simulink model "simulator_Force_Model"  (R2025b)
settings: Solver=FixedStepAuto  StartTime=0.0  StopTime=80  FixedStep=0.01  RelTol=1e-3
values from neighbouring files (symbols this model uses):
  dt = system_params.dt    [discretize_system.m]    (also in model_init.m)
  q0 = [0; 0; 0]    [model_init.m]    (also in test_model.m = x_test(1:3))
  qdot0 = [0;0;0]    [model_init.m]
undefined symbols (not defined in the file or in its folder): Cd, Dd, EKF_settings, P0, system_params, x0_EKF
libraries: slpidlib x5, mpclib x2
settings Model: Creator=Sigbjørn  LastModifiedBy=sig

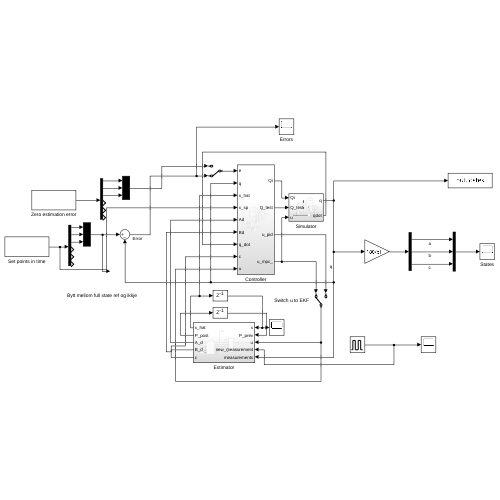
[thumbnail: Simulink's stored preview of the top-level diagram]
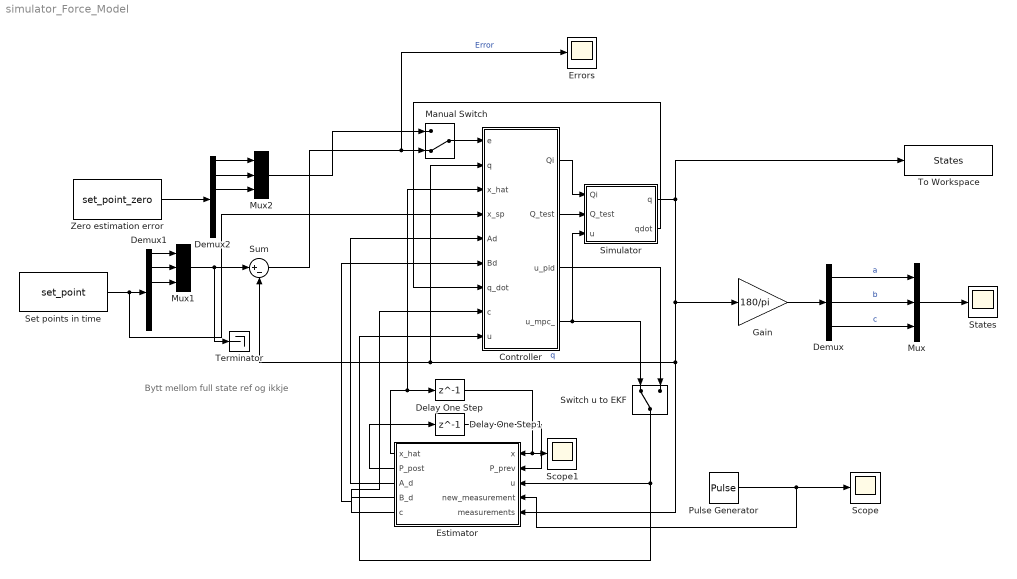
== system simulator_Force_Model ==
  note: Bytt mellom full state ref og ikkje
  Controller : Subsystem
  Delay One Step : Delay  DelayLength=1  InitialCondition=x0_EKF
  Delay One Step1 : Delay  DelayLength=1  InitialCondition=P0
  Demux : Demux  Outputs=3
  Demux1 : Demux  Outputs=6
  Demux2 : Demux  Outputs=6
  Errors : Scope
      settings: ActiveDisplayYMinimum=-1.818734816898053E+64  ActiveDisplayYMaximum=2.7677532819561327E+63
  Estimator : Subsystem
      settings: PortSchema="{\"entries\":[{\"content\":{\"sides\":[{\"content\":{\"connectorIds\":[\"Out1\",\"Out2\",\"Out3\",\"Out4\",\"Out5\"]},\"type\":\"ConnectorPlacement.EquallySpacedRectSide\",\"uuid\":\"f477ef40-4352-4d84-a45f-d7b8149414e1\"},{\"content\":{\"connectorIds\":[\"In1\",\"In2\",\"In3\",\"In4\",\"In5\"],\"side\":\"RIGHT\"},\"type\":\"ConnectorPlacement.EquallySpacedRectSide\",\"uuid\":\"8f29c47b-7819-47b7-a7db-3d460012710f\"},{\"content\":{\"side\":\"TOP\"},\"type\":\"ConnectorPlacement.EquallySpacedRectSide\",\"uuid\":\"6fcef62b-5cfa-49ba-93f4-5d540223ca0d\"}]},\"type\":\"ConnectorPlacement.EquallySpacedConnector\",\"uuid\":\"aa31ebfc-db05-4e23-be25-e9e271d34221\"}],\"packageUris\":[\"http://schema.mathworks.com/mf0/Connector/R2020b\"],\"version\":\"1.0\"}"
  Gain : Gain  Gain=180/pi
  Manual Switch : ManualSwitch  CurrentSetting=0
  Mux : Mux  Inputs=3
  Mux1 : Mux  Inputs=3
  Mux2 : Mux  Inputs=3
  Pulse Generator : DiscretePulseGenerator  PulseType=Time based  Period=0.02  PulseWidth=50
  Scope : Scope
      settings: ActiveDisplayYMinimum=-0.12120060790273554  ActiveDisplayYMaximum=1.1287993920972645  DataLoggingVariableName=ScopeData11
  Scope1 : Scope
      settings: ActiveDisplayYMinimum=-0.06497104688761951  ActiveDisplayYMaximum=0.02165522822111654  DataLoggingVariableName=ScopeData13
  Set points in time : FromWorkspace  VariableName=set_point
  Simulator : Subsystem
  States : Scope
      settings: ActiveDisplayYMinimum=-31.388895783470453  ActiveDisplayYMaximum=57.369364436172283
  Sum : Sum  Inputs=|+-
  Switch u to EKF : ManualSwitch
  Terminator : Terminator
  To Workspace : ToWorkspace  VariableName=States  SaveFormat=Timeseries  SampleTime=-1
  Zero estimation error : FromWorkspace  VariableName=set_point_zero
  wires:
  Controller/1(Qi) -> Simulator/1(Qi)
  Sum/1 -> Errors/1, Manual Switch/2  "Error"
  Simulator/1(q) -> To Workspace/1, Estimator/5(measurements), Sum/2, Controller/2(q), Gain/1  "q"
  Demux/1 -> Mux/1  "a"
  Demux/2 -> Mux/2  "b"
  Demux/3 -> Mux/3  "c"
  Manual Switch/1 -> Controller/1(e)
  Gain/1 -> Demux/1
  Mux/1 -> States/1
  Controller/2(Q_test) -> Simulator/2(Q_test)
  Pulse Generator/1 -> Estimator/4(new_measurement), Scope/1
  Estimator/2(P_post) -> Delay One Step1/1
  Delay One Step/1 -> Scope1/1, Estimator/1(x)
  Delay One Step1/1 -> Estimator/2(P_prev)
  Estimator/3(A_d) -> Controller/5(Ad)
  Estimator/4(B_d) -> Controller/6(Bd)
  Demux1/2 -> Mux1/2
  Demux1/1 -> Mux1/1
  Demux1/3 -> Mux1/3
  Mux1/1 -> Terminator/1, Sum/1
  Estimator/1(x_hat) -> Controller/3(x_hat), Delay One Step/1
  Demux2/3 -> Mux2/3
  Demux2/2 -> Mux2/2
  Zero estimation error/1 -> Demux2/1
  Demux2/1 -> Mux2/1
  Mux2/1 -> Manual Switch/1
  Simulator/2(qdot) -> Controller/7(q_dot)
  Estimator/5(c) -> Controller/8(c)
  Switch u to EKF/1 -> Estimator/3(u), Controller/9(u)
  Controller/4(u_mpc_) -> Switch u to EKF/1, Simulator/3(u)
  Controller/3(u_pid) -> Switch u to EKF/2
  Set points in time/1 -> Controller/4(x_sp), Demux1/1

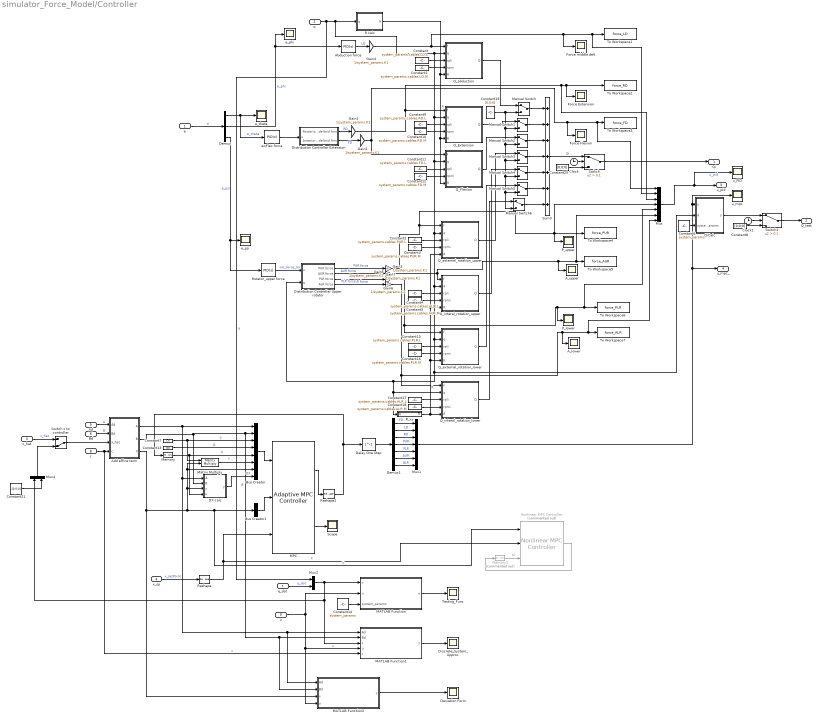
== system simulator_Force_Model/Controller ==
  e : Inport
  q : Inport  Port=2
  x_hat : Inport  Port=3
  x_sp : Inport  Port=4
  Ad : Inport  Port=5
  Bd : Inport  Port=6
  q_dot : Inport  Port=7
  c : Inport  Port=8
  u : Inport  Port=9
  A_lower : Scope
      settings: ActiveDisplayYMinimum=-66.70773  ActiveDisplayYMaximum=600.36959  DataLoggingVariableName=ScopeData3
  A_upper : Scope
      settings: ActiveDisplayYMinimum=-10.373094653487385  ActiveDisplayYMaximum=93.35785188138648  DataLoggingVariableName=ScopeData4
  Abduction force : slpidlib/PID Controller  Controller=PID  Form=Parallel  TimeDomain=Continuous-time  UseExternalTs=off  SampleTime=-1  IntegratorMethod=Forward Euler  FilterMethod=Forward Euler  ControllerParametersSource=internal  P=1  I=25  UseKiTs=off  D=5  UseExternalDerivativeSource=off  N=100  UseFilter=on  TunerSelectOption=Transfer Function Based (PID Tuner App)  InitialConditionSource=internal  InitialConditionForIntegrator=0  InitialConditionForFilter=0  DifferentiatorICPrevScaledInput=0  ExternalReset=none  TrackingMode=off  Kt=1  LimitOutput=on  SatLimitsSource=internal  UpperSaturationLimit=inf  LowerSaturationLimit=0  LinearizeAsGain=on  AntiWindupMode=none  Kb=1  LimitIntegrator=on  UpperIntegratorSaturationLimit=10000  LowerIntegratorSaturationLimit=0  POutMin=[]  POutMax=[]  IOutMin=[]  IOutMax=[]  DOutMin=[]  DOutMax=[]  NOutMin=[]  NOutMax=[]  SumOutMin=[]  SumOutMax=[]  SaturationOutMin=[]  SaturationOutMax=[]  PParamMin=[]  PParamMax=[]  IParamMin=[]  IParamMax=[]  DParamMin=[]  DParamMax=[]  NParamMin=[]  NParamMax=[]  KbParamMin=[]  KbParamMax=[]  KtParamMin=[]  KtParamMax=[]  KbOutMin=[]  KbOutMax=[]  KtOutMin=[]  KtOutMax=[]  IntegratorOutMin=[]  IntegratorOutMax=[]  FilterOutMin=[]  FilterOutMax=[]  SumI1OutMin=[]  SumI1OutMax=[]  SumI2OutMin=[]  SumI2OutMax=[]  SumI3OutMin=[]  SumI3OutMax=[]  SumI4OutMin=[]  SumI4OutMax=[]  SumDOutMin=[]  SumDOutMax=[]  DifferentiatorOutMin=[]  DifferentiatorOutMax=[]  FilterDiffOutCoefMin=[]  FilterDiffOutCoefMax=[]  ReciprocalOutMin=[]  ReciprocalOutMax=[]  SumDenOutMin=[]  SumDenOutMax=[]  SumNumOutMin=[]  SumNumOutMax=[]  DivideOutMin=[]  DivideOutMax=[]  UdiffTsProdOutMin=[]  UdiffTsProdOutMax=[]  NTsProdOutMin=[]  NTsProdOutMax=[]  UintegralTsProdOutMin=[]  UintegralTsProdOutMax=[]  UngainTsProdOutMin=[]  UngainTsProdOutMax=[]  ClampingZeroOutDataTypeStr=Inherit: Inherit via back propagation  ClampingZeroOutMin=[]  ClampingZeroOutMax=[]  FilterDenConstantOutDataTypeStr=Inherit: Inherit via back propagation  FilterDenConstantOutMin=[]  FilterDenConstantOutMax=[]  PCopyOutDataTypeStr=Inherit: Inherit via back propagation  PCopyOutMin=[]  PCopyOutMax=[]  NCopyOutDataTypeStr=Inherit: Inherit via back propagation  NCopyOutMin=[]  NCopyOutMax=[]  IntegratorContinuousStateAttributes=''  IntegratorStateMustResolveToSignalObject=off  IntegratorRTWStateStorageClass=Auto  FilterContinuousStateAttributes=''  FilterStateMustResolveToSignalObject=off  FilterRTWStateStorageClass=Auto  ParallelPVariant=InternalParameters  IdealPVariant=Disabled  IVariant=InternalParameters  DVariant=InternalParameters  IntegratorVariant=Continuous  SatVariant=Enabled  AWVariant=Passthrough  PCopyVariant=Disabled  TRVariant=Disabled  FdbkBlocksVariant=Forward  IdealPFdbkVariant=Disabled  SatFdbkVariant=Disabled  DerivativeFilterVariant=ContFilter  NVariant=InternalParameters  NCopyVariant=Disabled  FilterICVariant=InternalICsFilter  IntegratorICVariant=InternalICs  ExternalResetVariant=Disabled  TRSumVariant=Passthrough  SumFdbkVariant=Disabled  SumVariant=Sum_PID  TsampFilterVariant=InternalTs  TsampNgainVariant=Passthrough  TsampIntegralVariant=Disabled_SignalSpec  ExternalSaturationOutDataTypeStr=Inherit: Same as second input  DerivativeSourceVariant=ErrorSignal  PreIntVariant=InternalPreInt
  Add affine term : MATLAB Function  TreatAsAtomicUnit=on
  Bus Creator : BusCreator  Inputs=8
  Bus Creator1 : BusCreator  Inputs=1
  Clock : Clock
  Clock1 : Clock
  Constant : Constant  Value=system_params.cables.LD.L
  Constant1 : Constant  Value=system_params.cables.LD.M
  Constant10 : Constant  Value=system_params.cables.RD.M
  Constant11 : Constant  Value=system_params.cables.FD.L
  Constant12 : Constant  Value=system_params.cables.FD.M
  Constant13 : Constant  Value=Dd
  Constant14 : Constant  Value=system_params  OutDataTypeStr=Bus: System_params_bus
  Constant15 : Constant  Value=system_params.cables.PLR.L
  Constant16 : Constant  Value=system_params.cables.PLR.M
  Constant17 : Constant  Value=system_params.cables.ALR.L
  Constant18 : Constant  Value=system_params.cables.ALR.M
  Constant{8,19,21,25} (4 alike) : Constant  Value=[0;0;0]
  Constant2 : Constant  Value=system_params.cables.PUR.L
  Constant3 : Constant  Value=system_params.cables.PUR.M
  Constant4 : Constant  Value=system_params.cables.AUR.L
  Constant5 : Constant  Value=system_params.cables.AUR.M
  Constant6 : Constant  Value=system_params  OutDataTypeStr=Bus: System_params_bus
  Constant7 : Constant  Value=Cd
  Constant9 : Constant  Value=system_params.cables.RD.L
  DX calc : MATLAB Function  TreatAsAtomicUnit=on
  Delay One Step : Delay  DelayLength=1
  Demux : Demux  Outputs=3
  Demux1 : Demux  Outputs=7
  Deviation Form : Scope
      settings: ActiveDisplayYMinimum=-1  ActiveDisplayYMaximum=1  DataLoggingVariableName=ScopeData20
  Discrete_System_Approx : Scope
      settings: ActiveDisplayYMinimum=-0.51528443829155268  ActiveDisplayYMaximum=1.8768209864297223  DataLoggingVariableName=ScopeData18
  Distribution Controller Extension : Subsystem
  Distribution Controller Upper rotator : Subsystem
  Force Extension : Scope
      settings: ActiveDisplayYMinimum=-1.1404457548759319E-5  ActiveDisplayYMaximum=0.0001033020677424701
  Force Flexion : Scope
      settings: ActiveDisplayYMinimum=-0.00021802888941381923  ActiveDisplayYMaximum=0.0019628886422166426  DataLoggingVariableName=ScopeData2
  Force middle delt : Scope
      settings: ActiveDisplayYMinimum=-0.45342522545906838  ActiveDisplayYMaximum=4.0808270291316164  DataLoggingVariableName=ScopeData3
  Gain{1..7} (7 alike) : Gain  Gain=1/system_params.K1
  MATLAB Function : MATLAB Function  TreatAsAtomicUnit=on
  MATLAB Function1 : MATLAB Function  TreatAsAtomicUnit=on
  MATLAB Function2 : MATLAB Function  TreatAsAtomicUnit=on
  MPC : mpclib/Adaptive MPC Controller  SCDEnableBlockLinearizationSpecification=on  mpcobj=MPC_controller  enable_value=0  updateMPCinCallerWorkspace=on  md_inport=off  mv_inport=off  uref_inport=off  return_cost=on  return_mvseq=off  return_qpstatus=off  return_xseq=off  return_state=off  return_ovseq=off  state_inport=on  isltv_plant=off  umin_inport=off  umax_inport=off  ymin_inport=off  ymax_inport=off  cc_inport=off  ywt_inport=off  uwt_inport=off  duwt_inport=off  rhoeps_inport=off  pm_inport=off  MaximumP=10  HorizonChoice=FixedHorizon  BlockDataType=double  SampleTimeInherited=off  switch_inport=off
  Manual Switch{,1..6} (7 alike) : ManualSwitch
  Matrix Multiply : Product  Multiplication=Matrix(*)
  Memory : Memory  InitialCondition=[0;0;0;0;0;0;0]
  Memory1 : Memory  Commented=on  InitialCondition=[0;0;0;0;0;0;0]
  Mux : Mux  Inputs=7
  Mux1 : Mux  Inputs=7
  Mux2 : Mux  Inputs=2
  Mux4 : Mux  Inputs=2
  Nonlinear MPC Controller : mpclib/Nonlinear MPC Controller  Commented=on  nlmpcobj=NL_mpc  UseObjectTs=on  UseMEX=off  md_enabled=off  mvtarget_enabled=off  param_enabled=off  cost_enabled=off  mvseq_enabled=off  stateseq_enabled=off  ovseq_enabled=off  slack_enabled=off  status_enabled=off  ov_min=off  ov_max=off  mv_min=off  mv_max=off  mvrate_min=off  mvrate_max=off  state_min=off  state_max=off  ov_weight=off  mv_weight=off  mvrate_weight=off  ecr_weight=off  nlp_initialize=off
  P_lower : Scope
      settings: ActiveDisplayYMinimum=-3.51093  ActiveDisplayYMaximum=31.5984  DataLoggingVariableName=ScopeData2
  P_upper : Scope
      settings: ActiveDisplayYMinimum=-0.42649  ActiveDisplayYMaximum=3.83839
  Q_Extension : MATLAB Function  TreatAsAtomicUnit=on
  Q_Flexion : MATLAB Function  TreatAsAtomicUnit=on
  Q_abduction : MATLAB Function  TreatAsAtomicUnit=on
  Q_external_rotation_lower : MATLAB Function  TreatAsAtomicUnit=on
  Q_external_rotation_upper : MATLAB Function  TreatAsAtomicUnit=on
  Q_interal_rotation_lower : MATLAB Function  TreatAsAtomicUnit=on
  Q_interal_rotation_upper : MATLAB Function  TreatAsAtomicUnit=on
  QiCalc : MATLAB Function  TreatAsAtomicUnit=on
  R calc : MATLAB Function  TreatAsAtomicUnit=on
  R_xy : MATLAB Function  TreatAsAtomicUnit=on
  Reshape : Reshape  OutputDimensionality=Column vector (2-D)
  Reshape1 : Reshape  OutputDimensionality=Column vector (2-D)
  Rotator_upper force : slpidlib/PID Controller  Controller=PID  Form=Parallel  TimeDomain=Continuous-time  UseExternalTs=off  SampleTime=-1  IntegratorMethod=Forward Euler  FilterMethod=Forward Euler  ControllerParametersSource=internal  P=100  I=200  UseKiTs=off  D=500  UseExternalDerivativeSource=off  N=100  UseFilter=on  TunerSelectOption=Transfer Function Based (PID Tuner App)  InitialConditionSource=internal  InitialConditionForIntegrator=0  InitialConditionForFilter=0  DifferentiatorICPrevScaledInput=0  ExternalReset=none  TrackingMode=off  Kt=1  LimitOutput=on  SatLimitsSource=internal  UpperSaturationLimit=inf  LowerSaturationLimit=-inf  LinearizeAsGain=on  AntiWindupMode=none  Kb=1  LimitIntegrator=on  UpperIntegratorSaturationLimit=inf  LowerIntegratorSaturationLimit=-inf  POutMin=[]  POutMax=[]  IOutMin=[]  IOutMax=[]  DOutMin=[]  DOutMax=[]  NOutMin=[]  NOutMax=[]  SumOutMin=[]  SumOutMax=[]  SaturationOutMin=[]  SaturationOutMax=[]  PParamMin=[]  PParamMax=[]  IParamMin=[]  IParamMax=[]  DParamMin=[]  DParamMax=[]  NParamMin=[]  NParamMax=[]  KbParamMin=[]  KbParamMax=[]  KtParamMin=[]  KtParamMax=[]  KbOutMin=[]  KbOutMax=[]  KtOutMin=[]  KtOutMax=[]  IntegratorOutMin=[]  IntegratorOutMax=[]  FilterOutMin=[]  FilterOutMax=[]  SumI1OutMin=[]  SumI1OutMax=[]  SumI2OutMin=[]  SumI2OutMax=[]  SumI3OutMin=[]  SumI3OutMax=[]  SumI4OutMin=[]  SumI4OutMax=[]  SumDOutMin=[]  SumDOutMax=[]  DifferentiatorOutMin=[]  DifferentiatorOutMax=[]  FilterDiffOutCoefMin=[]  FilterDiffOutCoefMax=[]  ReciprocalOutMin=[]  ReciprocalOutMax=[]  SumDenOutMin=[]  SumDenOutMax=[]  SumNumOutMin=[]  SumNumOutMax=[]  DivideOutMin=[]  DivideOutMax=[]  UdiffTsProdOutMin=[]  UdiffTsProdOutMax=[]  NTsProdOutMin=[]  NTsProdOutMax=[]  UintegralTsProdOutMin=[]  UintegralTsProdOutMax=[]  UngainTsProdOutMin=[]  UngainTsProdOutMax=[]  ClampingZeroOutDataTypeStr=Inherit: Inherit via back propagation  ClampingZeroOutMin=[]  ClampingZeroOutMax=[]  FilterDenConstantOutDataTypeStr=Inherit: Inherit via back propagation  FilterDenConstantOutMin=[]  FilterDenConstantOutMax=[]  PCopyOutDataTypeStr=Inherit: Inherit via back propagation  PCopyOutMin=[]  PCopyOutMax=[]  NCopyOutDataTypeStr=Inherit: Inherit via back propagation  NCopyOutMin=[]  NCopyOutMax=[]  IntegratorContinuousStateAttributes=''  IntegratorStateMustResolveToSignalObject=off  IntegratorRTWStateStorageClass=Auto  FilterContinuousStateAttributes=''  FilterStateMustResolveToSignalObject=off  FilterRTWStateStorageClass=Auto  ParallelPVariant=InternalParameters  IdealPVariant=Disabled  IVariant=InternalParameters  DVariant=InternalParameters  IntegratorVariant=Continuous  SatVariant=Enabled  AWVariant=Passthrough  PCopyVariant=Disabled  TRVariant=Disabled  FdbkBlocksVariant=Forward  IdealPFdbkVariant=Disabled  SatFdbkVariant=Disabled  DerivativeFilterVariant=ContFilter  NVariant=InternalParameters  NCopyVariant=Disabled  FilterICVariant=InternalICsFilter  IntegratorICVariant=InternalICs  ExternalResetVariant=Disabled  TRSumVariant=Passthrough  SumFdbkVariant=Disabled  SumVariant=Sum_PID  TsampFilterVariant=InternalTs  TsampNgainVariant=Passthrough  TsampIntegralVariant=Disabled_SignalSpec  ExternalSaturationOutDataTypeStr=Inherit: Same as second input  DerivativeSourceVariant=ErrorSignal  PreIntVariant=InternalPreInt
  Scope : Scope
      settings: ActiveDisplayYMinimum=-740.0274786197964  ActiveDisplayYMaximum=6731.9872770462225  DataLoggingVariableName=ScopeData19
  Sum3 : Sum  Inputs=+++++++  InputSameDT=on  SaturateOnIntegerOverflow=on  OutDataTypeStr=Inherit: Same as first input
  Switch : Switch  Criteria=u2 > Threshold  Threshold=0.1  SaturateOnIntegerOverflow=off  InputSameDT=off
  Switch x to controller : ManualSwitch  CurrentSetting=0
  Switch1 : Switch  Criteria=u2 > Threshold  Threshold=0.1  SaturateOnIntegerOverflow=off  InputSameDT=off
  Testing_Func : Scope
      settings: ActiveDisplayYMinimum=-0.87802224801470286  ActiveDisplayYMaximum=2.0566387555111536  DataLoggingVariableName=ScopeData16
  To Workspace1 : ToWorkspace  VariableName=force_LD  SaveFormat=Timeseries  SampleTime=-1
  To Workspace2 : ToWorkspace  VariableName=force_RD  SaveFormat=Timeseries  SampleTime=-1
  To Workspace3 : ToWorkspace  VariableName=force_FD  SaveFormat=Timeseries  SampleTime=-1
  To Workspace4 : ToWorkspace  VariableName=force_PUR  SaveFormat=Timeseries  SampleTime=-1
  To Workspace5 : ToWorkspace  VariableName=force_AUR  SaveFormat=Timeseries  SampleTime=-1
  To Workspace6 : ToWorkspace  VariableName=force_PLR  SaveFormat=Timeseries  SampleTime=-1
  To Workspace7 : ToWorkspace  VariableName=force_ALR  SaveFormat=Timeseries  SampleTime=-1
  e_phi : Scope
      settings: ActiveDisplayYMinimum=-1  ActiveDisplayYMaximum=1  DataLoggingVariableName=ScopeData5
  e_psi : Scope
      settings: ActiveDisplayYMinimum=-0.000531028678053236  ActiveDisplayYMaximum=0.0043911774565179515  DataLoggingVariableName=ScopeData3
  e_theta : Scope
      settings: ActiveDisplayYMinimum=-0.0081249223165325481  ActiveDisplayYMaximum=0.0015822660919378819  DataLoggingVariableName=ScopeData6
  ex/flex force : slpidlib/PID Controller  Controller=PID  Form=Parallel  TimeDomain=Discrete-time  UseExternalTs=off  SampleTime=-1  IntegratorMethod=Forward Euler  FilterMethod=Forward Euler  ControllerParametersSource=internal  P=1  I=25  UseKiTs=off  D=5  UseExternalDerivativeSource=off  N=100  UseFilter=on  TunerSelectOption=Transfer Function Based (PID Tuner App)  InitialConditionSource=internal  InitialConditionForIntegrator=0  InitialConditionForFilter=0  DifferentiatorICPrevScaledInput=0  ExternalReset=none  TrackingMode=off  Kt=1  LimitOutput=on  SatLimitsSource=internal  UpperSaturationLimit=inf  LowerSaturationLimit=-inf  LinearizeAsGain=on  AntiWindupMode=none  Kb=1  LimitIntegrator=on  UpperIntegratorSaturationLimit=inf  LowerIntegratorSaturationLimit=-inf  POutMin=[]  POutMax=[]  IOutMin=[]  IOutMax=[]  DOutMin=[]  DOutMax=[]  NOutMin=[]  NOutMax=[]  SumOutMin=[]  SumOutMax=[]  SaturationOutMin=[]  SaturationOutMax=[]  PParamMin=[]  PParamMax=[]  IParamMin=[]  IParamMax=[]  DParamMin=[]  DParamMax=[]  NParamMin=[]  NParamMax=[]  KbParamMin=[]  KbParamMax=[]  KtParamMin=[]  KtParamMax=[]  KbOutMin=[]  KbOutMax=[]  KtOutMin=[]  KtOutMax=[]  IntegratorOutMin=[]  IntegratorOutMax=[]  FilterOutMin=[]  FilterOutMax=[]  SumI1OutMin=[]  SumI1OutMax=[]  SumI2OutMin=[]  SumI2OutMax=[]  SumI3OutMin=[]  SumI3OutMax=[]  SumI4OutMin=[]  SumI4OutMax=[]  SumDOutMin=[]  SumDOutMax=[]  DifferentiatorOutMin=[]  DifferentiatorOutMax=[]  FilterDiffOutCoefMin=[]  FilterDiffOutCoefMax=[]  ReciprocalOutMin=[]  ReciprocalOutMax=[]  SumDenOutMin=[]  SumDenOutMax=[]  SumNumOutMin=[]  SumNumOutMax=[]  DivideOutMin=[]  DivideOutMax=[]  UdiffTsProdOutMin=[]  UdiffTsProdOutMax=[]  NTsProdOutMin=[]  NTsProdOutMax=[]  UintegralTsProdOutMin=[]  UintegralTsProdOutMax=[]  UngainTsProdOutMin=[]  UngainTsProdOutMax=[]  ClampingZeroOutDataTypeStr=Inherit: Inherit via back propagation  ClampingZeroOutMin=[]  ClampingZeroOutMax=[]  FilterDenConstantOutDataTypeStr=Inherit: Inherit via back propagation  FilterDenConstantOutMin=[]  FilterDenConstantOutMax=[]  PCopyOutDataTypeStr=Inherit: Inherit via back propagation  PCopyOutMin=[]  PCopyOutMax=[]  NCopyOutDataTypeStr=Inherit: Inherit via back propagation  NCopyOutMin=[]  NCopyOutMax=[]  IntegratorContinuousStateAttributes=''  IntegratorStateMustResolveToSignalObject=off  IntegratorRTWStateStorageClass=Auto  FilterContinuousStateAttributes=''  FilterStateMustResolveToSignalObject=off  FilterRTWStateStorageClass=Auto  ParallelPVariant=InternalParameters  IdealPVariant=Disabled  IVariant=InternalParameters  DVariant=InternalParameters  IntegratorVariant=Discrete  SatVariant=Enabled  AWVariant=Passthrough  PCopyVariant=Disabled  TRVariant=Disabled  FdbkBlocksVariant=Forward  IdealPFdbkVariant=Disabled  SatFdbkVariant=Disabled  DerivativeFilterVariant=ForwardEulerFilter  NVariant=InternalParameters  NCopyVariant=Disabled  FilterICVariant=InternalICsFilter  IntegratorICVariant=InternalICs  ExternalResetVariant=Disabled  TRSumVariant=Passthrough  SumFdbkVariant=Disabled  SumVariant=Sum_PID  TsampFilterVariant=InternalTs  TsampNgainVariant=Passthrough  TsampIntegralVariant=Disabled_SignalSpec  ExternalSaturationOutDataTypeStr=Inherit: Same as second input  DerivativeSourceVariant=ErrorSignal  PreIntVariant=InternalPreInt
  u_PID : Scope
      settings: ActiveDisplayYMinimum=-0.0655807466436869  ActiveDisplayYMaximum=0.59022671979318231  DataLoggingVariableName=ScopeData15
  u_mpc : Scope
      settings: ActiveDisplayYMinimum=-0.10232300884956036  ActiveDisplayYMaximum=0.21294247787611242  DataLoggingVariableName=ScopeData14
  Qi : Outport
  Q_test : Outport  Port=2
  u_pid : Outport  Port=3
  u_mpc_ : Outport  Port=4
  wires:
  q/1 -> Mux2/1, Q_abduction/2(q), Q_Extension/2(q), Q_Flexion/2(q), QiCalc/2(q), Q_interal_rotation_lower/2(q), R_xy/1(q), Distribution Controller Upper rotator/2(q), Q_external_rotation_lower/2(q), Q_interal_rotation_upper/2(q), Q_external_rotation_upper/2(q), R calc/1(q)  "q"
  R calc/1(R) -> Q_Extension/5(R), Q_Flexion/5(R), Q_abduction/5(R)  "R"
  Constant/1 -> Q_abduction/3(rpli)
  Constant1/1 -> Q_abduction/4(rpmi)
  Sum3/1 -> Switch/1  "Qi"
  Demux/1 -> ex/flex force/1, e_theta/1  "e_theta"
  Demux/2 -> e_phi/1, Abduction force/1  "e_phi"
  Demux/3 -> Rotator_upper force/1, e_psi/1  "e_psi"
  Constant2/1 -> Q_external_rotation_upper/3(rpli)
  Constant3/1 -> Q_external_rotation_upper/4(rpmi)
  Constant4/1 -> Q_interal_rotation_upper/3(rpli)
  Constant5/1 -> Q_interal_rotation_upper/4(rpmi)
  Q_abduction/1(Q) -> Manual Switch/1
  Q_interal_rotation_upper/1(Q) -> Manual Switch4/1
  Q_external_rotation_upper/1(Q) -> Manual Switch3/1
  Rotator_upper force/1 -> Distribution Controller Upper rotator/1(u)  "rot_force_tot"
  ex/flex force/1 -> Distribution Controller Extension/1(u)
  Constant9/1 -> Q_Extension/3(rpli)
  Constant10/1 -> Q_Extension/4(rpmi)
  Constant11/1 -> Q_Flexion/3(rpli)
  Constant12/1 -> Q_Flexion/4(rpmi)
  Q_Flexion/1(Q) -> Manual Switch2/1
  Q_Extension/1(Q) -> Manual Switch1/1
  Abduction force/1 -> Gain4/1  "LD"
  Distribution Controller Extension/1(Posterior deltoid force) -> Gain1/1  "RD"
  Distribution Controller Extension/2(Anterior deltoid force) -> Gain2/1  "FD"
  Q_external_rotation_lower/1(Q) -> Manual Switch5/1
  Q_interal_rotation_lower/1(Q) -> Manual Switch6/1
  Constant15/1 -> Q_external_rotation_lower/3(rpli)
  Constant16/1 -> Q_external_rotation_lower/4(rpmi)
  Constant17/1 -> Q_interal_rotation_lower/3(rpli)
  Constant18/1 -> Q_interal_rotation_lower/4(rpmi)
  e/1 -> Demux/1  "e"
  Clock/1 -> Switch/2
  Constant25/1 -> Switch/3
  Switch/1 -> Qi/1
  Distribution Controller Upper rotator/4(ALR force) -> Gain7/1  "ALR force"
  Distribution Controller Upper rotator/3(PLR force) -> Gain6/1  "PLR force"
  Distribution Controller Upper rotator/2(AUR force) -> Gain5/1  "AUR force"
  Distribution Controller Upper rotator/1(PUR force) -> Gain3/1  "PUR force"
  R_xy/1(R) -> Q_external_rotation_upper/5(R), Q_interal_rotation_upper/5(R), Q_external_rotation_lower/5(R), Q_interal_rotation_lower/5(R)  "R"
  Mux/1 -> u_PID/1, u_pid/1  "u_pid"
  QiCalc/1(y) -> Switch1/1
  Constant6/1 -> QiCalc/3(system_params)
  Ad/1 -> Add affine term/1(Ad)  "A"
  Add affine term/2(B) -> MATLAB Function1/2(Bd), MATLAB Function2/2(Bd), Bus Creator/2, DX calc/2(B)  "B"
  x_sp/1 -> Reshape/1  "x_setPoint"
  Constant8/1 -> Switch1/3
  Switch1/1 -> Q_test/1
  Clock1/1 -> Switch1/2
  MPC/1 -> Reshape1/1
  Bus Creator/1 -> MPC/1
  Bus Creator1/1 -> MPC/2
  Constant7/1 -> Bus Creator/3, Matrix Multiply/1  "C"
  Constant13/1 -> Bus Creator/4  "D"
  Matrix Multiply/1 -> Bus Creator/6  "Y"
  DX calc/1(y) -> Bus Creator/8  "DX"
  Reshape1/1 -> Memory/1, Delay One Step/1
  Demux1/7 -> Mux1/7  "ALR"
  Demux1/6 -> Mux1/6  "AUR"
  Demux1/5 -> Mux1/5  "PLR"
  Demux1/4 -> Mux1/4  "PUR"
  Demux1/3 -> Mux1/3  "RD"
  Demux1/2 -> Mux1/2  "LD"
  Demux1/1 -> Mux1/1  "FD"
  MATLAB Function/1(y) -> Testing_Func/1
  q_dot/1 -> Mux2/2  "q_dot"
  Constant14/1 -> MATLAB Function/3(system_params)
  MATLAB Function1/1(y) -> Discrete_System_Approx/1
  Constant19/1 -> Manual Switch3/2, Manual Switch4/2, Manual Switch5/2, Manual Switch6/2, Manual Switch2/2, Manual Switch1/2, Manual Switch/2
  c/1 -> MATLAB Function1/5(c), Add affine term/4(c)  "c"
  MATLAB Function2/1(y) -> Deviation Form/1
  Mux2/1 -> Mux4/1, MATLAB Function1/3(x), MATLAB Function/1(x)
  Add affine term/3(X) -> MATLAB Function2/3(x), Nonlinear MPC Controller/1, Bus Creator1/1, DX calc/3(x), Bus Creator/7, Matrix Multiply/2  "X"
  Memory/1 -> DX calc/4(u), Bus Creator/5  "U"
  Reshape/1 -> Nonlinear MPC Controller/2, MPC/3  "X"
  Add affine term/1(A) -> MATLAB Function1/1(Ad), MATLAB Function2/1(Ad), DX calc/1(A), Bus Creator/1
  Bd/1 -> Add affine term/2(Bd)  "B"
  x_hat/1 -> Switch x to controller/1  "x_hat"
  Mux1/1 -> u_mpc_/1, QiCalc/1(u), u_mpc/1
  Delay One Step/1 -> Demux1/1
  Switch x to controller/1 -> Add affine term/3(x_hat)
  u/1 -> MATLAB Function2/4(u), MATLAB Function1/4(u), MATLAB Function/2(u)  "u"
  Constant21/1 -> Mux4/2
  Mux4/1 -> Switch x to controller/2
  Manual Switch/1 -> Sum3/1
  Manual Switch1/1 -> Sum3/2
  Manual Switch2/1 -> Sum3/3
  Manual Switch3/1 -> Sum3/4
  Manual Switch4/1 -> Sum3/5
  Manual Switch5/1 -> Sum3/6
  Manual Switch6/1 -> Sum3/7
  Gain4/1 -> Q_abduction/1(f), Force middle delt/1, Mux/2, To Workspace1/1
  Gain1/1 -> Mux/3, To Workspace2/1, Force Extension/1, Q_Extension/1(f)
  Gain2/1 -> Q_Flexion/1(f), Mux/1, To Workspace3/1, Force Flexion/1
  Gain3/1 -> Mux/4, To Workspace4/1, P_upper/1, Q_external_rotation_upper/1(f)
  Gain5/1 -> A_upper/1, Mux/6, To Workspace5/1, Q_interal_rotation_upper/1(f)
  Gain6/1 -> Mux/5, To Workspace6/1, P_lower/1, Q_external_rotation_lower/1(f)
  Gain7/1 -> Mux/7, To Workspace7/1, A_lower/1, Q_interal_rotation_lower/1(f)
  MPC/2 -> Scope/1
  Nonlinear MPC Controller/1 -> Memory1/1
  Memory1/1 -> Nonlinear MPC Controller/3  "U"

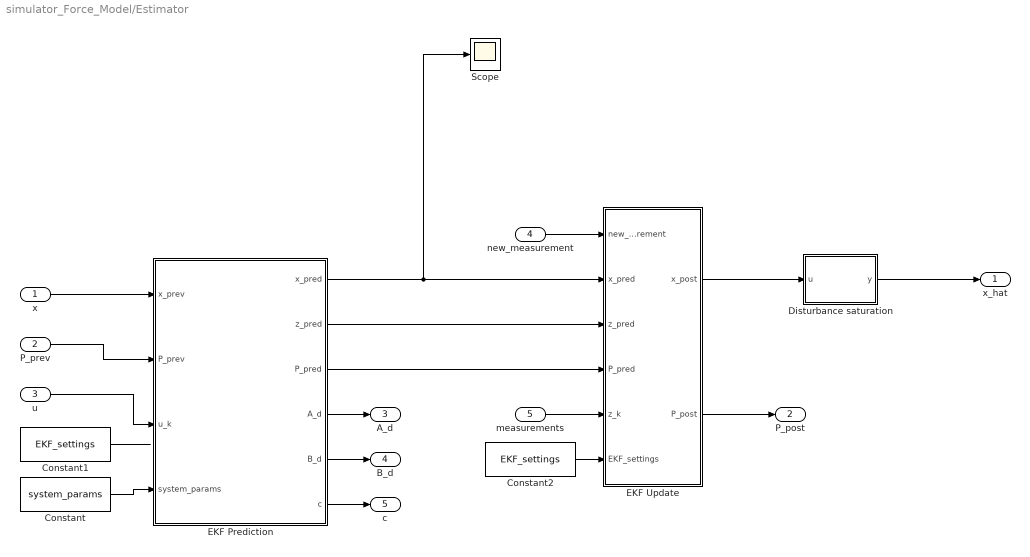
== system simulator_Force_Model/Estimator ==
  x : Inport
  P_prev : Inport  Port=2
  u : Inport  Port=3
  new_measurement : Inport  Port=4
  measurements : Inport  Port=5
  Constant : Constant  Value=system_params  OutDataTypeStr=Bus: System_params_bus
  Constant1 : Constant  Value=EKF_settings  OutDataTypeStr=Bus: EKFBus
  Constant2 : Constant  Value=EKF_settings  OutDataTypeStr=Bus: EKFBus
  Disturbance saturation : MATLAB Function  TreatAsAtomicUnit=on
  EKF Prediction : MATLAB Function  TreatAsAtomicUnit=on
  EKF Update : MATLAB Function  TreatAsAtomicUnit=on
  Scope : Scope
      settings: ActiveDisplayYMinimum=-1  ActiveDisplayYMaximum=1  DataLoggingVariableName=ScopeData12
  x_hat : Outport
  P_post : Outport  Port=2
  A_d : Outport  Port=3
  B_d : Outport  Port=4
  c : Outport  Port=5
  wires:
  x/1 -> EKF Prediction/1(x_prev)
  EKF Update/1(x_post) -> Disturbance saturation/1(u)
  u/1 -> EKF Prediction/3(u_k)
  P_prev/1 -> EKF Prediction/2(P_prev)
  Constant/1 -> EKF Prediction/4(system_params)
  EKF Prediction/1(x_pred) -> Scope/1, EKF Update/2(x_pred)
  EKF Prediction/2(z_pred) -> EKF Update/3(z_pred)
  EKF Prediction/3(P_pred) -> EKF Update/4(P_pred)
  EKF Prediction/4(A_d) -> A_d/1
  EKF Prediction/5(B_d) -> B_d/1
  new_measurement/1 -> EKF Update/1(new_measurement)
  EKF Update/2(P_post) -> P_post/1
  measurements/1 -> EKF Update/5(z_k)
  EKF Prediction/6(c) -> c/1
  Constant1/1 -> ?
  Constant2/1 -> EKF Update/6(EKF_settings)
  Disturbance saturation/1(y) -> x_hat/1

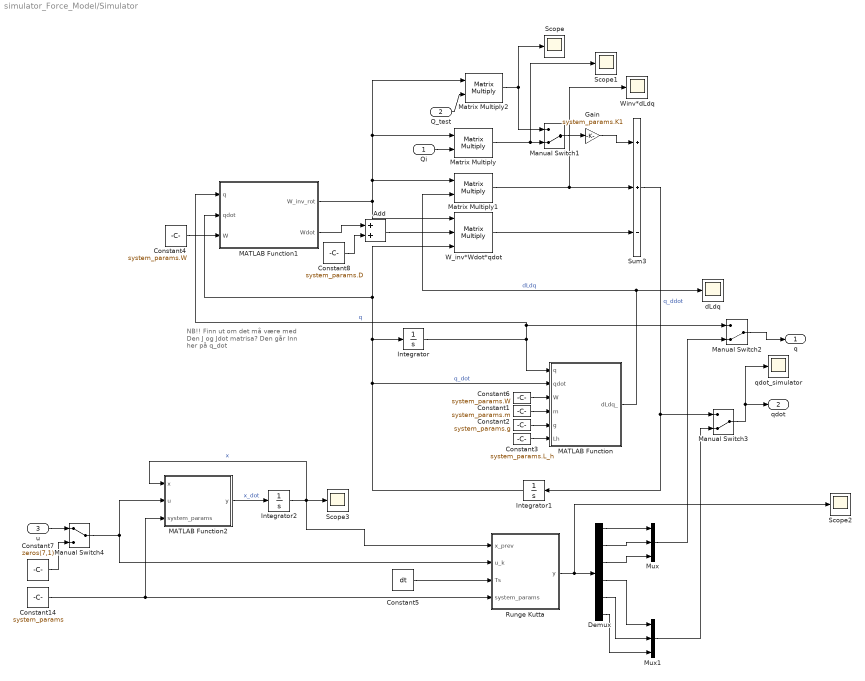
== system simulator_Force_Model/Simulator ==
  note: NB!! Finn ut om det må være med
      | Den J og Jdot matrisa? Den går
      | Inn her på q_dot
  Qi : Inport
  Q_test : Inport  Port=2
  u : Inport  Port=3
  Add : Sum
  Constant1 : Constant  Value=system_params.m
  Constant14 : Constant  Value=system_params  OutDataTypeStr=Bus: System_params_bus
  Constant2 : Constant  Value=system_params.g
  Constant3 : Constant  Value=system_params.L_h
  Constant4 : Constant  Value=system_params.W
  Constant5 : Constant  Value=dt
  Constant6 : Constant  Value=system_params.W
  Constant7 : Constant  Value=zeros(7,1)
  Constant8 : Constant  Value=system_params.D
  Demux : Demux  Outputs=6
  Gain : Gain  Gain=system_params.K1
  Integrator : Integrator  InitialCondition=q0
  Integrator1 : Integrator  InitialCondition=qdot0
  Integrator2 : Integrator  InitialCondition=[q0;qdot0]
  MATLAB Function : MATLAB Function  TreatAsAtomicUnit=on
  MATLAB Function1 : MATLAB Function  TreatAsAtomicUnit=on
  MATLAB Function2 : MATLAB Function  TreatAsAtomicUnit=on
  Manual Switch1 : ManualSwitch  CurrentSetting=0
  Manual Switch2 : ManualSwitch  CurrentSetting=0
  Manual Switch3 : ManualSwitch  CurrentSetting=0
  Manual Switch4 : ManualSwitch
  Matrix Multiply : Product  Multiplication=Matrix(*)
  Matrix Multiply1 : Product  Multiplication=Matrix(*)
  Matrix Multiply2 : Product  Multiplication=Matrix(*)
  Mux : Mux  Inputs=3
  Mux1 : Mux  Inputs=3
  Runge Kutta : MATLAB Function  TreatAsAtomicUnit=on
  Scope{,1..3} (4 alike) : Scope
      Scope settings: ActiveDisplayYMinimum=-12.627932166058498  ActiveDisplayYMaximum=18.695188809418351  DataLoggingVariableName=ScopeData9
      Scope1 settings: ActiveDisplayYMinimum=-3.4678856908682762  ActiveDisplayYMaximum=14.936630459412994  DataLoggingVariableName=ScopeData10
      Scope2 settings: ActiveDisplayYMinimum=-1.2516190957732058  ActiveDisplayYMaximum=1.2509215238841511  DataLoggingVariableName=ScopeData21
      Scope3 settings: ActiveDisplayYMinimum=-2.7543101989253471  ActiveDisplayYMaximum=1.0721408599751914  DataLoggingVariableName=ScopeData22
  Sum3 : Sum  Inputs=++-  InputSameDT=on  SaturateOnIntegerOverflow=on  OutDataTypeStr=Inherit: Same as first input
  W_inv*Wdot*qdot : Product  Inputs=3  Multiplication=Matrix(*)
  Winv*dLdq : Scope
      settings: ActiveDisplayYMinimum=-1  ActiveDisplayYMaximum=1
  dLdq : Scope
      settings: ActiveDisplayYMinimum=-0.79665266597510709  ActiveDisplayYMaximum=0.68877686845714259  DataLoggingVariableName=ScopeData2
  qdot_simulator : Scope
      settings: ActiveDisplayYMinimum=-0.26387984719349139  ActiveDisplayYMaximum=0.31183044301786966  DataLoggingVariableName=ScopeData17
  q : Outport
  qdot : Outport  Port=2
  wires:
  Qi/1 -> Matrix Multiply/2
  Constant1/1 -> MATLAB Function/4(m)
  Constant2/1 -> MATLAB Function/5(g)
  Constant3/1 -> MATLAB Function/6(Lh)
  Integrator/1 -> Manual Switch2/1, MATLAB Function1/1(q), MATLAB Function/1(q)  "q"
  Integrator1/1 -> W_inv*Wdot*qdot/3, MATLAB Function1/2(qdot), Integrator/1, MATLAB Function/2(qdot)  "q_dot"
  MATLAB Function/1(dLdq_) -> dLdq/1, Matrix Multiply1/2  "dLdq"
  Sum3/1 -> Manual Switch3/1, Integrator1/1  "q_ddot"
  Matrix Multiply/1 -> Manual Switch1/2, Scope1/1
  Matrix Multiply1/1 -> Winv*dLdq/1, Sum3/2
  MATLAB Function1/2(Wdot) -> Add/1
  MATLAB Function1/1(W_inv_rot) -> Matrix Multiply2/1, Matrix Multiply/1, Matrix Multiply1/1, W_inv*Wdot*qdot/1
  Constant4/1 -> MATLAB Function1/3(W)
  W_inv*Wdot*qdot/1 -> Sum3/3
  Constant6/1 -> MATLAB Function/3(W)
  Matrix Multiply2/1 -> Manual Switch1/1, Scope/1
  Q_test/1 -> Matrix Multiply2/2
  Manual Switch1/1 -> Gain/1
  Gain/1 -> Sum3/1
  Manual Switch2/1 -> q/1
  Constant14/1 -> MATLAB Function2/3(system_params), Runge Kutta/4(system_params)
  Constant5/1 -> Runge Kutta/3(Ts)
  u/1 -> Manual Switch4/1
  Runge Kutta/1(y) -> Scope2/1, Demux/1
  Demux/1 -> Mux/1
  Demux/2 -> Mux/2
  Demux/3 -> Mux/3
  Demux/4 -> Mux1/1
  Demux/5 -> Mux1/2
  Demux/6 -> Mux1/3
  Mux/1 -> Manual Switch2/2
  Mux1/1 -> Manual Switch3/2
  Manual Switch3/1 -> qdot/1, qdot_simulator/1
  Manual Switch4/1 -> MATLAB Function2/2(u), Runge Kutta/2(u_k)
  Constant7/1 -> Manual Switch4/2
  MATLAB Function2/1(y) -> Integrator2/1  "x_dot"
  Integrator2/1 -> Runge Kutta/1(x_prev), Scope3/1, MATLAB Function2/1(x)  "x"
  Add/1 -> W_inv*Wdot*qdot/2
  Constant8/1 -> Add/2

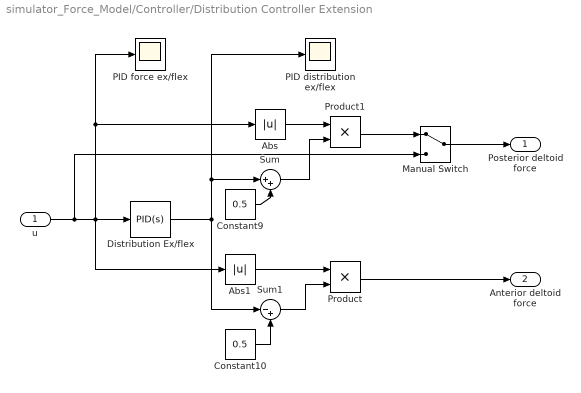
== system simulator_Force_Model/Controller/Distribution Controller Extension ==
  u : Inport
  Abs : Abs  SaturateOnIntegerOverflow=off
  Abs1 : Abs  SaturateOnIntegerOverflow=off
  Constant10 : Constant  Value=0.5
  Constant9 : Constant  Value=0.5
  Distribution Ex/flex : slpidlib/PID Controller  Controller=PID  Form=Parallel  TimeDomain=Continuous-time  UseExternalTs=off  SampleTime=-1  IntegratorMethod=Forward Euler  FilterMethod=Forward Euler  ControllerParametersSource=internal  P=100  I=0  UseKiTs=off  D=0  UseExternalDerivativeSource=off  N=100  UseFilter=on  TunerSelectOption=Transfer Function Based (PID Tuner App)  InitialConditionSource=internal  InitialConditionForIntegrator=0  InitialConditionForFilter=0  DifferentiatorICPrevScaledInput=0  ExternalReset=none  TrackingMode=off  Kt=1  LimitOutput=on  SatLimitsSource=internal  UpperSaturationLimit=0.45  LowerSaturationLimit=-0.45  LinearizeAsGain=on  AntiWindupMode=none  Kb=1  LimitIntegrator=on  UpperIntegratorSaturationLimit=10  LowerIntegratorSaturationLimit=0  POutMin=[]  POutMax=[]  IOutMin=[]  IOutMax=[]  DOutMin=[]  DOutMax=[]  NOutMin=[]  NOutMax=[]  SumOutMin=[]  SumOutMax=[]  SaturationOutMin=[]  SaturationOutMax=[]  PParamMin=[]  PParamMax=[]  IParamMin=[]  IParamMax=[]  DParamMin=[]  DParamMax=[]  NParamMin=[]  NParamMax=[]  KbParamMin=[]  KbParamMax=[]  KtParamMin=[]  KtParamMax=[]  KbOutMin=[]  KbOutMax=[]  KtOutMin=[]  KtOutMax=[]  IntegratorOutMin=[]  IntegratorOutMax=[]  FilterOutMin=[]  FilterOutMax=[]  SumI1OutMin=[]  SumI1OutMax=[]  SumI2OutMin=[]  SumI2OutMax=[]  SumI3OutMin=[]  SumI3OutMax=[]  SumI4OutMin=[]  SumI4OutMax=[]  SumDOutMin=[]  SumDOutMax=[]  DifferentiatorOutMin=[]  DifferentiatorOutMax=[]  FilterDiffOutCoefMin=[]  FilterDiffOutCoefMax=[]  ReciprocalOutMin=[]  ReciprocalOutMax=[]  SumDenOutMin=[]  SumDenOutMax=[]  SumNumOutMin=[]  SumNumOutMax=[]  DivideOutMin=[]  DivideOutMax=[]  UdiffTsProdOutMin=[]  UdiffTsProdOutMax=[]  NTsProdOutMin=[]  NTsProdOutMax=[]  UintegralTsProdOutMin=[]  UintegralTsProdOutMax=[]  UngainTsProdOutMin=[]  UngainTsProdOutMax=[]  ClampingZeroOutDataTypeStr=Inherit: Inherit via back propagation  ClampingZeroOutMin=[]  ClampingZeroOutMax=[]  FilterDenConstantOutDataTypeStr=Inherit: Inherit via back propagation  FilterDenConstantOutMin=[]  FilterDenConstantOutMax=[]  PCopyOutDataTypeStr=Inherit: Inherit via back propagation  PCopyOutMin=[]  PCopyOutMax=[]  NCopyOutDataTypeStr=Inherit: Inherit via back propagation  NCopyOutMin=[]  NCopyOutMax=[]  IntegratorContinuousStateAttributes=''  IntegratorStateMustResolveToSignalObject=off  IntegratorRTWStateStorageClass=Auto  FilterContinuousStateAttributes=''  FilterStateMustResolveToSignalObject=off  FilterRTWStateStorageClass=Auto  ParallelPVariant=InternalParameters  IdealPVariant=Disabled  IVariant=InternalParameters  DVariant=InternalParameters  IntegratorVariant=Continuous  SatVariant=Enabled  AWVariant=Passthrough  PCopyVariant=Disabled  TRVariant=Disabled  FdbkBlocksVariant=Forward  IdealPFdbkVariant=Disabled  SatFdbkVariant=Disabled  DerivativeFilterVariant=ContFilter  NVariant=InternalParameters  NCopyVariant=Disabled  FilterICVariant=InternalICsFilter  IntegratorICVariant=InternalICs  ExternalResetVariant=Disabled  TRSumVariant=Passthrough  SumFdbkVariant=Disabled  SumVariant=Sum_PID  TsampFilterVariant=InternalTs  TsampNgainVariant=Passthrough  TsampIntegralVariant=Disabled_SignalSpec  ExternalSaturationOutDataTypeStr=Inherit: Same as second input  DerivativeSourceVariant=ErrorSignal  PreIntVariant=InternalPreInt
  Manual Switch : ManualSwitch
  PID distribution ex/flex : Scope
      settings: ActiveDisplayYMinimum=-0.5625  ActiveDisplayYMaximum=0.5625  DataLoggingVariableName=ScopeData8
  PID force ex/flex : Scope
      settings: ActiveDisplayYMinimum=-0.16319  ActiveDisplayYMaximum=0.10006  DataLoggingVariableName=ScopeData7
  Product : Product
  Product1 : Product
  Sum : Sum  Inputs=|++
  Sum1 : Sum  Inputs=|-+
  Posterior deltoid force : Outport
  Anterior deltoid force : Outport  Port=2
  wires:
  Constant10/1 -> Sum1/2
  u/1 -> Manual Switch/2, Distribution Ex/flex/1, PID force ex/flex/1, Abs/1, Abs1/1
  Distribution Ex/flex/1 -> Sum1/1, PID distribution ex/flex/1, Sum/1
  Abs1/1 -> Product/1
  Sum/1 -> Product1/2
  Sum1/1 -> Product/2
  Abs/1 -> Product1/1
  Constant9/1 -> Sum/2
  Product1/1 -> Manual Switch/1
  Product/1 -> Anterior deltoid force/1
  Manual Switch/1 -> Posterior deltoid force/1

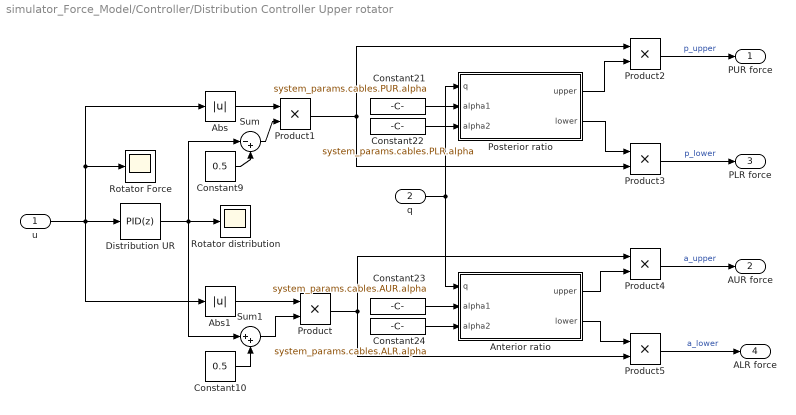
== system simulator_Force_Model/Controller/Distribution Controller Upper rotator ==
  u : Inport
  q : Inport  Port=2
  Abs : Abs  SaturateOnIntegerOverflow=off
  Abs1 : Abs  SaturateOnIntegerOverflow=off
  Anterior ratio : MATLAB Function  TreatAsAtomicUnit=on
  Constant10 : Constant  Value=0.5
  Constant21 : Constant  Value=system_params.cables.PUR.alpha
  Constant22 : Constant  Value=system_params.cables.PLR.alpha
  Constant23 : Constant  Value=system_params.cables.AUR.alpha
  Constant24 : Constant  Value=system_params.cables.ALR.alpha
  Constant9 : Constant  Value=0.5
  Distribution UR : slpidlib/PID Controller  Controller=PID  Form=Parallel  TimeDomain=Discrete-time  UseExternalTs=off  SampleTime=-1  IntegratorMethod=Forward Euler  FilterMethod=Forward Euler  ControllerParametersSource=internal  P=100  I=0  UseKiTs=off  D=0  UseExternalDerivativeSource=off  N=100  UseFilter=on  TunerSelectOption=Transfer Function Based (PID Tuner App)  InitialConditionSource=internal  InitialConditionForIntegrator=0  InitialConditionForFilter=0  DifferentiatorICPrevScaledInput=0  ExternalReset=none  TrackingMode=off  Kt=1  LimitOutput=on  SatLimitsSource=internal  UpperSaturationLimit=0.45  LowerSaturationLimit=-0.45  LinearizeAsGain=on  AntiWindupMode=none  Kb=1  LimitIntegrator=on  UpperIntegratorSaturationLimit=10  LowerIntegratorSaturationLimit=0  POutMin=[]  POutMax=[]  IOutMin=[]  IOutMax=[]  DOutMin=[]  DOutMax=[]  NOutMin=[]  NOutMax=[]  SumOutMin=[]  SumOutMax=[]  SaturationOutMin=[]  SaturationOutMax=[]  PParamMin=[]  PParamMax=[]  IParamMin=[]  IParamMax=[]  DParamMin=[]  DParamMax=[]  NParamMin=[]  NParamMax=[]  KbParamMin=[]  KbParamMax=[]  KtParamMin=[]  KtParamMax=[]  KbOutMin=[]  KbOutMax=[]  KtOutMin=[]  KtOutMax=[]  IntegratorOutMin=[]  IntegratorOutMax=[]  FilterOutMin=[]  FilterOutMax=[]  SumI1OutMin=[]  SumI1OutMax=[]  SumI2OutMin=[]  SumI2OutMax=[]  SumI3OutMin=[]  SumI3OutMax=[]  SumI4OutMin=[]  SumI4OutMax=[]  SumDOutMin=[]  SumDOutMax=[]  DifferentiatorOutMin=[]  DifferentiatorOutMax=[]  FilterDiffOutCoefMin=[]  FilterDiffOutCoefMax=[]  ReciprocalOutMin=[]  ReciprocalOutMax=[]  SumDenOutMin=[]  SumDenOutMax=[]  SumNumOutMin=[]  SumNumOutMax=[]  DivideOutMin=[]  DivideOutMax=[]  UdiffTsProdOutMin=[]  UdiffTsProdOutMax=[]  NTsProdOutMin=[]  NTsProdOutMax=[]  UintegralTsProdOutMin=[]  UintegralTsProdOutMax=[]  UngainTsProdOutMin=[]  UngainTsProdOutMax=[]  ClampingZeroOutDataTypeStr=Inherit: Inherit via back propagation  ClampingZeroOutMin=[]  ClampingZeroOutMax=[]  FilterDenConstantOutDataTypeStr=Inherit: Inherit via back propagation  FilterDenConstantOutMin=[]  FilterDenConstantOutMax=[]  PCopyOutDataTypeStr=Inherit: Inherit via back propagation  PCopyOutMin=[]  PCopyOutMax=[]  NCopyOutDataTypeStr=Inherit: Inherit via back propagation  NCopyOutMin=[]  NCopyOutMax=[]  IntegratorContinuousStateAttributes=''  IntegratorStateMustResolveToSignalObject=off  IntegratorRTWStateStorageClass=Auto  FilterContinuousStateAttributes=''  FilterStateMustResolveToSignalObject=off  FilterRTWStateStorageClass=Auto  ParallelPVariant=InternalParameters  IdealPVariant=Disabled  IVariant=InternalParameters  DVariant=InternalParameters  IntegratorVariant=Discrete  SatVariant=Enabled  AWVariant=Passthrough  PCopyVariant=Disabled  TRVariant=Disabled  FdbkBlocksVariant=Forward  IdealPFdbkVariant=Disabled  SatFdbkVariant=Disabled  DerivativeFilterVariant=ForwardEulerFilter  NVariant=InternalParameters  NCopyVariant=Disabled  FilterICVariant=InternalICsFilter  IntegratorICVariant=InternalICs  ExternalResetVariant=Disabled  TRSumVariant=Passthrough  SumFdbkVariant=Disabled  SumVariant=Sum_PID  TsampFilterVariant=InternalTs  TsampNgainVariant=Passthrough  TsampIntegralVariant=Disabled_SignalSpec  ExternalSaturationOutDataTypeStr=Inherit: Same as second input  DerivativeSourceVariant=ErrorSignal  PreIntVariant=InternalPreInt
  Posterior ratio : MATLAB Function  TreatAsAtomicUnit=on
  Product{,1..5} (6 alike) : Product
  Rotator Force : Scope
      settings: ActiveDisplayYMinimum=-13.1342  ActiveDisplayYMaximum=118.2078  DataLoggingVariableName=ScopeData5
  Rotator distribution : Scope
  Sum : Sum  Inputs=|-+
  Sum1 : Sum  Inputs=|++
  PUR force : Outport
  AUR force : Outport  Port=2
  PLR force : Outport  Port=3
  ALR force : Outport  Port=4
  wires:
  Constant10/1 -> Sum1/2
  u/1 -> Abs1/1, Distribution UR/1, Rotator Force/1, Abs/1
  Distribution UR/1 -> Rotator distribution/1, Sum1/1, Sum/1
  Abs1/1 -> Product/1
  Sum/1 -> Product1/2
  Sum1/1 -> Product/2
  Abs/1 -> Product1/1
  Constant9/1 -> Sum/2
  Posterior ratio/1(upper) -> Product2/2
  Constant24/1 -> Anterior ratio/3(alpha2)
  Constant23/1 -> Anterior ratio/2(alpha1)
  Anterior ratio/2(lower) -> Product5/1
  Product5/1 -> ALR force/1  "a_lower"
  q/1 -> Posterior ratio/1(q), Anterior ratio/1(q)
  Constant21/1 -> Posterior ratio/2(alpha1)
  Constant22/1 -> Posterior ratio/3(alpha2)
  Anterior ratio/1(upper) -> Product4/2
  Product/1 -> Product4/1, Product5/2
  Product2/1 -> PUR force/1  "p_upper"
  Posterior ratio/2(lower) -> Product3/1
  Product4/1 -> AUR force/1  "a_upper"
  Product1/1 -> Product3/2, Product2/1
  Product3/1 -> PLR force/1  "p_lower"

== matlab function simulator_Force_Model/Controller/R_xy ==
  data: q input; R output
function R = fcn(q)
R = Rot_xy(q);

== matlab function simulator_Force_Model/Controller/Q_external_rotation_lower ==
  data: f input; Q output; q input; rpli input; rpmi input; R input
function Q = fcn(f, q, rpli, rpmi, R)

Q = Qi(f, q, rpli, rpmi, R);

== matlab function simulator_Force_Model/Controller/Q_interal_rotation_lower ==
  data: f input; Q output; q input; rpli input; rpmi input; R input
function Q = fcn(f, q, rpli, rpmi, R)

Q = Qi(f, q, rpli, rpmi, R);

== matlab function simulator_Force_Model/Controller/QiCalc ==
  settings: updateMethod=DISCRETE  sampleTime=dt
  data: u input; y output; q input; system_params input
function y = fcn(u,q,system_params)
y = Q_force_calc(u, q, system_params);

== matlab function simulator_Force_Model/Estimator/EKF Prediction ==
  data: x_prev input; x_pred output; P_prev input; u_k input; z_pred output; P_pred output; A_d output; B_d output; system_params input; c output; EKF_settings parameter
function [x_pred, z_pred, P_pred, A_d, B_d, c] = fcn(x_prev, P_prev, u_k, system_params, EKF_settings)

[x_pred, z_pred, P_pred, A_d, B_d, c] = EKF_pred(x_prev, P_prev, u_k, EKF_settings, system_params);

== matlab function simulator_Force_Model/Controller/Distribution Controller Upper rotator/Anterior ratio ==
  data: q input; upper output; alpha1 input; alpha2 input; lower output
function [upper, lower] = ul_rat(q, alpha1, alpha2)

[upper, lower] = ul_ratio(q, alpha1, alpha2);

== matlab function simulator_Force_Model/Controller/Distribution Controller Upper rotator/Posterior ratio ==
  data: q input; upper output; alpha1 input; alpha2 input; lower output
function [upper, lower] = ul_rat(q, alpha1, alpha2)

[upper, lower] = ul_ratio(q, alpha1, alpha2);

== matlab function simulator_Force_Model/Estimator/EKF Update ==
  data: new_measurement input; x_pred input; z_pred input; x_post output; P_pred input; z_k input; EKF_settings input; P_post output
function [x_post,P_post] = fcn(new_measurement, x_pred, z_pred, P_pred, z_k, EKF_settings)
persistent isInitialized
if isempty(isInitialized)
    x_pred = EKF_settings.x0;
    P_pred = EKF_settings.P0;
    isInitialized = true;
end

if new_measurement
    [x_post,P_post] = EKF_upd(x_pred, P_pred, z_pred, z_k, EKF_settings);
else
    x_post = x_pred;
    P_post = P_pred;
end

== matlab function simulator_Force_Model/Simulator/MATLAB Function1 ==
  data: q input; qdot input; W input; W_inv_rot output; Wdot output
function [W_inv_rot, Wdot] = W_Wdot_call(q, qdot, W)

[W_inv_rot, Wdot] = W_Wdot(q, qdot, W);

== matlab function simulator_Force_Model/Controller/DX calc ==
  data: A input; B input; x input; u input; y output
function y = fcn(A,B,x,u)
y = A*x + B*u - x;

== matlab function simulator_Force_Model/Controller/MATLAB Function ==
  data: x input; u input; y output; system_params input
function y = fcn(x,u,system_params)
%y = system_model_continous(x, u, system_params);
y = runge_kutta4(x, u, 0.01, system_params);

== matlab function simulator_Force_Model/Controller/MATLAB Function1 ==
  data: Ad input; Bd input; x input; u input; y output; c input
function y = fcn(Ad,Bd,x,u,c)
Ad = Ad(1:6,1:6);
Bd = Bd(1:6,1:7);
c = c(1:6);
y = Ad*x + Bd*u + c;

== matlab function simulator_Force_Model/Controller/MATLAB Function2 ==
  data: Ad input; Bd input; x input; u input; y output
function y = fcn(Ad,Bd,x,u)
%x = [x;1];
y = Ad*x + Bd*u;
%y = Ad*x + Bd*u;

== matlab function simulator_Force_Model/Controller/Add affine term ==
  data: Ad input double; A output; Bd input; x_hat input; B output; X output; c input
function [A,B,X] = fcn(Ad,Bd,x_hat,c)
A = [Ad c; zeros(1,size(Ad,1)) 0];
B = [Bd; zeros(1,size(Bd,2))];
X = [x_hat;1];

== matlab function simulator_Force_Model/Estimator/Disturbance saturation ==
  data: u input; y output
function y = fcn(u)
lLim = -0.1;
uLim = 0.1;

for i=7:9
    if u(i) > uLim
        u(i) = uLim;
    elseif u(i) < lLim
        u(i) = lLim;
    end
end
y = u;

== matlab function simulator_Force_Model/Simulator/MATLAB Function2 ==
  data: x input; u input; y output; system_params input
function y = fcn(x, u, system_params)

y = system_model_continous(x, u, system_params);

== matlab function simulator_Force_Model/Simulator/Runge Kutta ==
  data: x_prev input; y output; u_k input; Ts input; system_params input
function y = fcn(x_prev, u_k, Ts, system_params)
y = runge_kutta4(x_prev, u_k, Ts, system_params);

== matlab function simulator_Force_Model/Simulator/MATLAB Function ==
  data: q input; qdot input; W input; dLdq_ output; m input; g input; Lh input
function dLdq_ = dLdq_call(q, qdot, W, m, g, Lh)
    temp_struct.W = W;
    temp_struct.m = m;
    temp_struct.g = g;
    temp_struct.L_h = Lh;
    dLdq_ = dLdq(q, qdot, temp_struct);
end

== matlab function simulator_Force_Model/Controller/R calc ==
  data: q input; R output
function R = fcn(q)
R = Rot_mat(q);

== matlab function simulator_Force_Model/Controller/Q_abduction ==
  data: f input; Q output; q input; rpli input; rpmi input; R input
function Q = fcn(f, q, rpli, rpmi, R)

Q = Qi(f, q, rpli, rpmi, R);

== matlab function simulator_Force_Model/Controller/Q_external_rotation_upper ==
  data: f input; Q output; q input; rpli input; rpmi input; R input
function Q = fcn(f, q, rpli, rpmi, R)

Q = Qi(f, q, rpli, rpmi, R);

== matlab function simulator_Force_Model/Controller/Q_interal_rotation_upper ==
  data: f input; Q output; q input; rpli input; rpmi input; R input
function Q = fcn(f, q, rpli, rpmi, R)

Q = Qi(f, q, rpli, rpmi, R);

== matlab function simulator_Force_Model/Controller/Q_Extension ==
  data: f input; Q output; q input; rpli input; rpmi input; R input
function Q = fcn(f, q, rpli, rpmi, R)

Q = Qi(f, q, rpli, rpmi, R);

== matlab function simulator_Force_Model/Controller/Q_Flexion ==
  data: f input; Q output; q input; rpli input; rpmi input; R input
function Q = fcn(f, q, rpli, rpmi, R)

Q = Qi(f, q, rpli, rpmi, R);
